simulink model "y5s"  (R2023b)
settings: Solver=FixedStepAuto  StartTime=0.0  StopTime=100  FixedStep=0.01  RelTol=1e-3
model workspace (MAT data in the model file):
  a1 = 1
  a2 = 1
  g = 9.8
  k = 20
  k2 = Simulink.Parameter
  k2.DataType = 'auto'
  k2.Complexity = 'real'
  k2.Dimensions = [0 0]
  m = 100
settings Model: Creator=asus  LastModifiedBy=asus

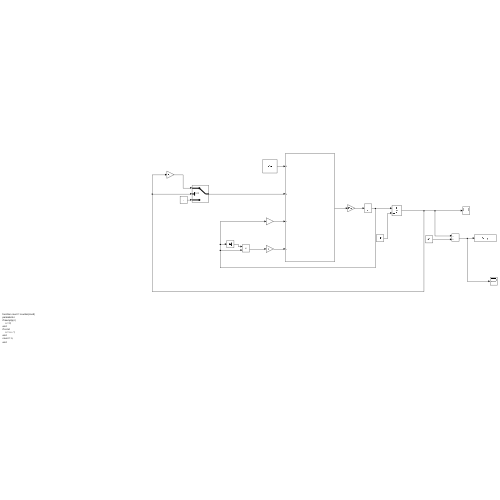
[thumbnail: Simulink's stored preview of the top-level diagram]
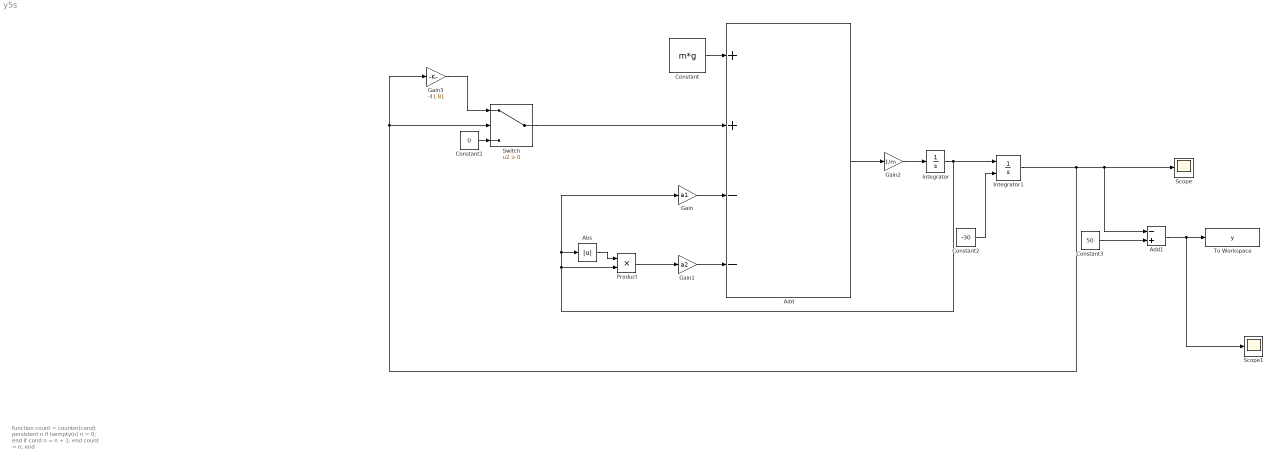
== system y5s ==
  note: function count = counter(cond)
      | persistent n
      | if isempty(n)
      |     n = 0;
      | end
      | if cond
      |     n = n + 1;
      | end
      | count = n;
      | end
  Abs : Abs  SaturateOnIntegerOverflow=off
  Add : Sum  Inputs=++--
  Add1 : Sum  Inputs=-+
  Constant : Constant  Value=m*g
  Constant1 : Constant  Value=0
  Constant2 : Constant  Value=-30
  Constant3 : Constant  Value=50
  Gain : Gain  Gain=a1
  Gain1 : Gain  Gain=a2
  Gain2 : Gain  Gain=1/m
  Gain3 : Gain  Gain=-41.81
  Integrator : Integrator
  Integrator1 : Integrator  InitialConditionSource=external  InitialCondition=-30
  Product : Product
  Scope : Scope
  Scope1 : Scope
  Switch : Switch  Criteria=u2 > Threshold  SaturateOnIntegerOverflow=off  InputSameDT=off
  To Workspace : ToWorkspace  VariableName=y  SampleTime=-1
  wires:
  Constant/1 -> Add/1
  Gain/1 -> Add/3
  Gain1/1 -> Add/4
  Add/1 -> Gain2/1
  Gain2/1 -> Integrator/1
  Integrator/1 -> Product/2, Gain/1, Abs/1, Integrator1/1
  Product/1 -> Gain1/1
  Abs/1 -> Product/1
  Switch/1 -> Add/2
  Integrator1/1 -> Add1/1, Scope/1, Gain3/1, Switch/2
  Constant1/1 -> Switch/3
  Constant2/1 -> Integrator1/2
  Constant3/1 -> Add1/2
  Add1/1 -> Scope1/1, To Workspace/1
  Gain3/1 -> Switch/1
